simulink model "taketwo_v1"  (R2024a)
settings: Solver=FixedStepAuto  StartTime=0.0  StopTime=100  FixedStep=0.05  RelTol=1e-3
libraries: robotlib x5
settings Model: Creator=katiegildersleeve  LastModifiedBy=katiegildersleeve
settings OptimizationCC: EnhancedBackFolding=on  PassReuseOutputArgsAs=Individual arguments  ZeroExternalMemoryAtStartup=off  ZeroInternalMemoryAtStartup=off  MaxStackSize=64  OptimizeBlockOrder=speed  DifferentSizesBufferReuse=on  OptimizationCustomize=off  EfficientTunableParamExpr=on
settings DebuggingCC: ParameterTunabilityLossMsg=error
settings HardwareCC: ProdBitPerPointer=32  ProdBitPerSizeT=32  ProdBitPerPtrDiffT=32  ProdLargestAtomicFloat=None  ProdIntDivRoundTo=Undefined  ProdEndianess=Unspecified  ProdWordSize=32  ProdHWDeviceType=Generic->Unspecified (assume 32-bit Generic)
settings SFSimCC: MATLABDynamicMemAlloc=off
settings RTWCC: Description=Embedded Coder  SystemTargetFile=ert.tlc  HardwareBoard=Robot Operating System (ROS)  TLCOptions="-aInlineSetEventsForThisBaseRateFcn=TLC_FALSE -aSuppressMultiTaskScheduler=TLC_FALSE  -aRateBasedStepFcn=0"  GenCodeOnly=on  TemplateMakefile=ert_default_tmf  Toolchain=Catkin  TargetLang=C++
settings CodeAppCC: ForceParamTrailComments=on  IgnoreCustomStorageClasses=off  OperatorAnnotations=on  SimulinkDataObjDesc=on  SFDataObjDesc=on  InsertBlockDesc=on

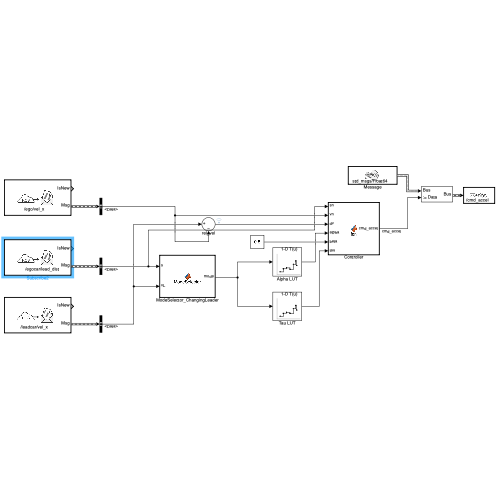
[thumbnail: Simulink's stored preview of the top-level diagram]
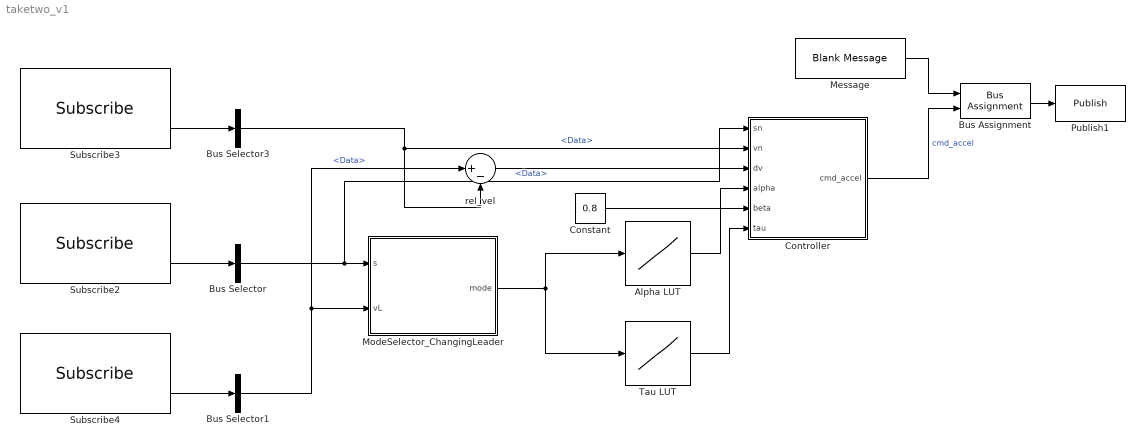
== system taketwo_v1 ==
  Alpha LUT : Lookup_n-D  NumberOfTableDimensions=1  BreakpointsForDimension1=[0 1 2 3]  Table=[0.75 0.75 1.0 0.25]  InterpMethod=Nearest  InternalRulePriority=Speed  RndMeth=Simplest
  Bus Assignment : BusAssignment  AssignedSignals=Data
  Bus Selector : BusSelector  OutputSignals=Data
  Bus Selector1 : BusSelector  OutputSignals=Data
  Bus Selector3 : BusSelector  OutputSignals=Data
  Constant : Constant  Value=0.8
  Controller : MATLAB Function  TreatAsAtomicUnit=on
  Message : robotlib/Blank Message  messageClass=Message  entityType=std_msgs/Float64  messageType=std_msgs/Float64  SampleTime=inf  legacyBusStruct=off
  ModeSelector_ChangingLeader : MATLAB Function  TreatAsAtomicUnit=on
  Publish1 : robotlib/Publish  topicSource=Specify your own  topic=/cmd_accel  messageType=std_msgs/Float64  legacyBusStruct=off  messageQueueLength=1
  Subscribe2 : robotlib/Subscribe  topicSource=Specify your own  topic=/egocar/lead_dist  messageType=std_msgs/Float64  SampleTime=0.05  legacyBusStruct=off  messageQueueLength=1
  Subscribe3 : robotlib/Subscribe  topicSource=Specify your own  topic=/ego/vel_x  messageType=std_msgs/Float64  SampleTime=0.05  legacyBusStruct=off  messageQueueLength=1
  Subscribe4 : robotlib/Subscribe  topicSource=Specify your own  topic=/leadcar/vel_x  messageType=std_msgs/Float64  SampleTime=0.05  legacyBusStruct=off  messageQueueLength=1
  Tau LUT : Lookup_n-D  NumberOfTableDimensions=1  BreakpointsForDimension1=[0 1 2 3]  Table=[0.75 0.75 0.5 3.0]  InterpMethod=Nearest  InternalRulePriority=Speed  RndMeth=Simplest
  rel_vel : Sum  Inputs=|+-
  wires:
  Tau LUT/1 -> Controller/6(tau)
  rel_vel/1 -> Controller/3(dv)
  ModeSelector_ChangingLeader/1(mode) -> Tau LUT/1, Alpha LUT/1
  Constant/1 -> Controller/5(beta)
  Alpha LUT/1 -> Controller/4(alpha)
  Subscribe2/2 -> Bus Selector/1
  Bus Selector/1 -> Controller/1(sn), ModeSelector_ChangingLeader/1(s)  "<Data>"
  Subscribe4/2 -> Bus Selector1/1
  Bus Selector1/1 -> rel_vel/1, ModeSelector_ChangingLeader/2(vL)  "<Data>"
  Bus Assignment/1 -> Publish1/1
  Message/1 -> Bus Assignment/1
  Controller/1(cmd_accel) -> Bus Assignment/2  "cmd_accel"
  Bus Selector3/1 -> rel_vel/2, Controller/2(vn)  "<Data>"
  Subscribe3/2 -> Bus Selector3/1

== matlab function taketwo_v1/Controller ==
  data: sn input; vn input; dv input; cmd_accel output; alpha input; beta input; tau input
function cmd_accel = fcn(sn, vn, dv, alpha, beta, tau)
% sn   : geometric gap (lead back - ego front) [m]
% vn   : ego speed [m/s]
% dv   : v_lead - v_ego [m/s]   (NEG when ego is faster)

    % ---- force scalars in case any input arrives as a vector ----
    sn    = double(sn(1));
    vn    = double(vn(1));
    dv    = double(dv(1));
    alpha = double(alpha(1));
    beta  = double(beta(1));
    tau   = double(tau(1));

    % --- constants ---
    s_min = 5.0;     % standstill buffer [m]
    s_far = 50.0;    % use cruise control when gap > this [m]
    v_des = 25.0;    % desired cruise speed [m/s]
    a_min = -3.0;    % max braking  [m/s^2]
    a_max =  1.5;    % max accel    [m/s^2]

    % predeclare to fix output dimension
    a = 0.0;

    if sn > s_far
        % Far from leader: simple speed hold
        a = beta .* (v_des - vn);
    else
        % Within 50 m: time-gap + relative-velocity PD
        sn_eff = max(sn - s_min, 0.0);
        a = alpha .* (sn_eff - tau .* vn) + beta .* dv;

        % Emergency rule: inside buffer and still closing -> full brake
        if sn <= s_min && dv < 0
            a = a_min;
        end
    end

    % Clamp to actuator limits
    cmd_accel = min(max(a, a_min), a_max);
end

== matlab function taketwo_v1/ModeSelector_ChangingLeader ==
  settings: updateMethod=DISCRETE
  data: s input; mode output; vL input
function mode = ModeSelector(s, vL)
% 1 = no leader (s>50)
% 2 = collecting (warm-up)
% 3 = smooth leader (after warm-up)
% 4 = erratic leader (after warm-up)

%#codegen
% ---------- Tunables ----------
Ts               = 0.05;   % match model fixed-step
S_NOLEADER       = 50.0;   % [m]
COLLECT_SECS     = 15.0;   % [s]
S_JUMP_THR       = 15.0;   % [m]
EWMA_TAU         = 3.0;    % [s]
SIGMA_LOW        = 0.50;   % [m/s]
SIGMA_HIGH       = 0.80;   % [m/s]
% --------------------------------

persistent inited prev_s prev_present collect_cnt mu var last_mode
if isempty(inited)
    inited        = true;
    prev_s        = s;
    prev_present  = (s <= S_NOLEADER);
    % *** Force warm-up if a leader is present at t=0 ***
    collect_cnt   = int32( prev_present * round(COLLECT_SECS / Ts) );
    mu            = vL;
    var           = 0.0;
    last_mode     = uint8(1);
end

leader_present = (s <= S_NOLEADER);

% (A) start warm-up when leader first appears (no->yes)
if leader_present && ~prev_present
    collect_cnt = int32(round(COLLECT_SECS / Ts));
    mu = vL; var = 0.0;
end

% (B) restart warm-up on any large one-sample space-gap jump
ds = s - prev_s;
if abs(ds) >= S_JUMP_THR
    collect_cnt = int32(round(COLLECT_SECS / Ts));
    mu = vL; var = 0.0;
end

% EWMA update only when leader present
alpha = Ts / max(EWMA_TAU, Ts); if alpha > 1, alpha = 1; end
if leader_present
    mu  = (1 - alpha)*mu + alpha*vL;
    d   = vL - mu;
    var = (1 - alpha)*(var + alpha*d*d);
else
    mu = vL; var = 0.0;
end
sigma = sqrt(max(var,0.0));

% ----- Mode decision -----
if ~leader_present
    mode = uint8(1);
else
    if collect_cnt > 0
        collect_cnt = collect_cnt - 1;
        mode = uint8(2);              % *** hold Mode 2 during warm-up ***
    else
        % hysteresis classification after warm-up
        if last_mode == uint8(4)
            mode = uint8( sigma <= SIGMA_LOW ) * 3 + uint8( sigma > SIGMA_LOW ) * 4;
        else
            mode = uint8( sigma >= SIGMA_HIGH ) * 4 + uint8( sigma < SIGMA_HIGH ) * 3;
        end
    end
end

% Bookkeeping
last_mode    = mode;
prev_s       = s;
prev_present = leader_present;
